simulink model "pvgrid"  (Simulink 7.8)
settings: Solver=ode23t  StartTime=0.0  StopTime=0.15  RelTol=1e-3
libraries: powerlib x15, powerlib_extras x5, simulink x1
settings Model: Creator=Administrator  LastModifiedBy=shinesong
settings OptimizationCC: InitFltsAndDblsToZero=on
settings DebuggingCC: FcnCallInpInsideContextMsg=Use local settings  StrictBusMsg=Warning

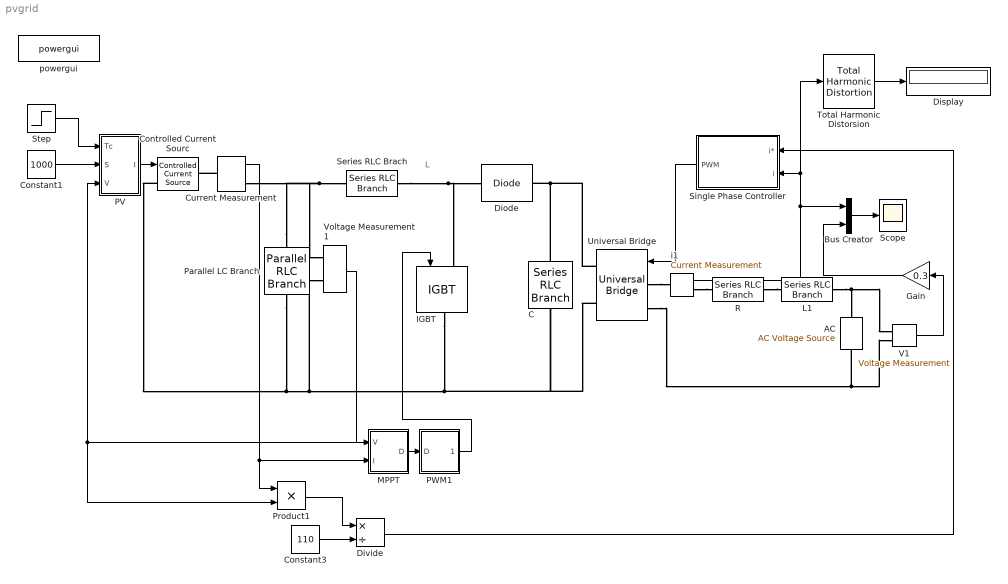
== system pvgrid ==
  note: L
  AC : powerlib/Electrical Sources/AC Voltage Source  Amplitude=155.5  Phase=0  Frequency=60  SampleTime=0  Measurements=None
  Bus Creator : BusCreator  Inputs=2
  C : powerlib/Elements/Series RLC Branch  LConnTagsString=__new0  RConnTagsString=__new0  BranchType=C  Resistance=1.0  Inductance=1.0  SetiL0=off  InitialCurrent=0  Capacitance=22e-6  Setx0=off  InitialVoltage=0  Measurements=None
  Constant1 : Constant  Value=1000
  Constant3 : Constant  Value=110
  Controlled Current Sourc : powerlib/Electrical Sources/Controlled Current Source  Initialize=on  Source_Type=DC  Amplitude=0  Phase=0  Frequency=0  Measurements=None
  Current Measurement : powerlib/Measurements/Current Measurement  PhasorSimulation=off  OutputType=Complex  PSBequivalent=0
  Diode : powerlib/Power Electronics/Diode  Ron=0.001  Lon=0  Vf=0.8  IC=0  UseSnubber=off  Rs=500  Cs=250e-9  Measurements=off
  Display : Display
  Divide : Product  Inputs=*/
  Gain : Gain  Gain=0.3
  IGBT : powerlib/Power Electronics/IGBT  Ron=0.001  Lon=0  Vf=1  Tf=1e-6  Tt=2e-6  IC=0  Rs=1e5  Cs=inf  Measurements=off
  L1 : powerlib/Elements/Series RLC Branch  LConnTagsString=__new0  RConnTagsString=__new0  BranchType=L  Resistance=1.0  Inductance=2e-2  SetiL0=off  InitialCurrent=0  Capacitance=1.0  Setx0=off  InitialVoltage=0  Measurements=None
  MPPT : Subsystem
  PV : Subsystem  mask{Im=13.88, Vm=281.6, Voc=353.6, Isc=14.88, Sref=1000, Tref=25, a=0.015, b=0.7, Rs=2}
      mask help: PV_modle
  PWM1 : Subsystem  mask{Ts=0.00001, Fs=5e4}
      mask prompts: Ts "Sample Time"; Fs "Frequency of Tri Wave"
  Parallel LC Branch : powerlib/Elements/Parallel RLC Branch  LConnTagsString=a  RConnTagsString=__new0  BranchType=C  Resistance=1.0  Inductance=1.0  SetiL0=off  InitialCurrent=0  Capacitance=110e-6  Setx0=off  InitialVoltage=0  Measurements=None
  Product1 : Product  RndMeth=Zero
  R : powerlib/Elements/Series RLC Branch  LConnTagsString=__new0  RConnTagsString=__new0  BranchType=R  Resistance=0.01  Inductance=10e-3  SetiL0=off  InitialCurrent=0  Capacitance=1.0  Setx0=off  InitialVoltage=0  Measurements=None
  Scope : Scope
      settings: YMin=2.5  YMax=35
  Series RLC Brach : powerlib/Elements/Series RLC Branch  LConnTagsString=__new0  RConnTagsString=__new0  BranchType=L  Resistance=1.0  Inductance=150e-6  SetiL0=off  InitialCurrent=0  Capacitance=1.0  Setx0=off  InitialVoltage=0  Measurements=None
  Single Phase Controller : Subsystem
  Step : Step  Time=0.1  Before=25  After=85  SampleTime=0
  Total Harmonic Distorsion : powerlib_extras/Measurements/Total Harmonic Distortion  f1=60
  Universal Bridge : powerlib/Power Electronics/Universal Bridge  Arms=2  SnubberResistance=1e5  SnubberCapacitance=inf  Device=MOSFET / Diodes  Ron=1e-3  Lon=0  ForwardVoltages="[  0  0  ]"  ForwardVoltage=0  GTOparameters=[ 10e-6 , 20e-6 ]  IGBTparameters=[ 1e-6 , 2e-6 ]  Measurements=None  Measurements_2=None  converterType=Rectifier
  V1 : powerlib/Measurements/Voltage Measurement  PhasorSimulation=off  OutputType=Complex  PSBequivalent=0
  Voltage Measurement1 : powerlib/Measurements/Voltage Measurement  PhasorSimulation=off  OutputType=Complex  PSBequivalent=0
  i1 : powerlib/Measurements/Current Measurement  PhasorSimulation=off  OutputType=Complex  PSBequivalent=0
  powergui : powerlib/powergui  SimulationMode=Discrete  SolverType=Tustin  SampleTime=5e-7  frequency=60  SPID=off  DisableSnubberDevices=off  DisableRonSwitches=off  DisableVfSwitches=off  SwTol=0  Interpol=off  DisplayEquations=off  FunctionMessages=off  frequencyindice=60  Pbase=100e6  ErrMax=1e-4  Iterations=50  UnitsV=kV  UnitsW=MW  echomessages=off  HookPort=off  EnableUseOfTLC=off  x0status=blocks  RestoreLinks=warning  ResistiveCurrentMeasurement=off  Frange=[0:2:500]  Ylog=off  Xlog=on  ShowGrid=off  save=off  variable=ZData  structure=ScopeData5  ZoomFFT=off  StartTime=0.0  cycles=1  DisplayStyle=1  fundamental=60  FreqAxis=off  MaxFrequency=1000  frequencyindicesteady=1  RmsSteady=1  display=off  Ts=0  methode=off
  wires:
  Single Phase Controller/1(PWM) -> Universal Bridge/1
  i1/1 -> Bus Creator/1, Single Phase Controller/2(i), Total Harmonic Distorsion/1
  Product1/1 -> Divide/1
  Voltage Measurement1/1 -> Product1/2, PV/3(V), MPPT/1(V)
  Constant3/1 -> Divide/2
  Divide/1 -> Single Phase Controller/1(i*)
  Bus Creator/1 -> Scope/1
  PV/1(I) -> Controlled Current Sourc/1
  Step/1 -> PV/1(Tc)
  MPPT/1(D) -> PWM1/1(D)
  Total Harmonic Distorsion/1 -> Display/1
  Current Measurement/1 -> Product1/1, MPPT/2(I)
  PWM1/1(pwm) -> IGBT/1
  Constant1/1 -> PV/2(S)
  V1/1 -> Gain/1
  Gain/1 -> Bus Creator/2
  connections:
  Universal Bridge/LConn1 -- i1/LConn1
  i1/RConn1 -- R/LConn1
  R/RConn1 -- L1/LConn1
  Universal Bridge/LConn2 -- AC/LConn1 -- V1/LConn2
  L1/RConn1 -- AC/RConn1 -- V1/LConn1
  Parallel LC Branch/LConn1 -- Current Measurement/RConn1 -- Voltage Measurement1/LConn1 -- Series RLC Brach/LConn1
  Series RLC Brach/RConn1 -- IGBT/LConn1 -- Diode/LConn1
  C/RConn1 -- IGBT/RConn1 -- Controlled Current Sourc/LConn1 -- Parallel LC Branch/RConn1 -- Voltage Measurement1/LConn2 -- Universal Bridge/RConn2
  C/LConn1 -- Diode/RConn1 -- Universal Bridge/RConn1
  Current Measurement/LConn1 -- Controlled Current Sourc/RConn1

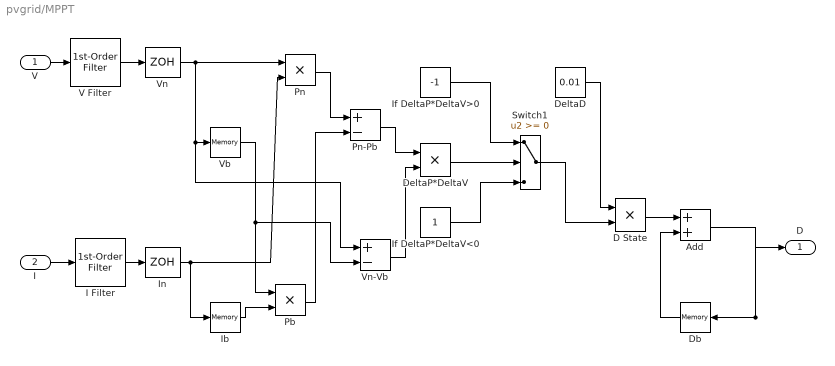
== system pvgrid/MPPT ==
  V : Inport
  I : Inport  Port=2
  Add : Sum
  D State : Product  RndMeth=Zero
  Db : Memory  InheritSampleTime=on  LinearizeAsDelay=on
  DeltaD : Constant  Value=0.01
  DeltaP*DeltaV : Product  RndMeth=Zero
  I Filter : powerlib_extras/Control  Blocks/1st-Order  Filter  FilterType=Lowpass  Tc=1e-3  Initialize=off  Vac_Init=[0.8 -25 60]  Vdc_Init=-0.4  PlotResponse=off  param1=[1 500 1]
  Ib : Memory  InheritSampleTime=on  LinearizeAsDelay=on
  If DeltaP*DeltaV<0 : Constant
  If DeltaP*DeltaV>0 : Constant  Value=-1
  In : ZeroOrderHold  SampleTime=1e-4
  Pb : Product  RndMeth=Zero
  Pn : Product  RndMeth=Zero
  Pn-Pb : Sum  Inputs=+-
  Switch1 : Switch
  V Filter : powerlib_extras/Control  Blocks/1st-Order  Filter  FilterType=Lowpass  Tc=1e-3  Initialize=off  Vac_Init=[0.8 -25 60]  Vdc_Init=-0.4  PlotResponse=off  param1=[1 500 1]
  Vb : Memory  InheritSampleTime=on  LinearizeAsDelay=on
  Vn : ZeroOrderHold  SampleTime=1e-4
  Vn-Vb : Sum  Inputs=+-
  D : Outport
  wires:
  V/1 -> V Filter/1
  I/1 -> I Filter/1
  V Filter/1 -> Vn/1
  I Filter/1 -> In/1
  In/1 -> Ib/1, Pn/2
  Vn/1 -> Pn/1, Vb/1, Vn-Vb/1
  Ib/1 -> Pb/2
  Vb/1 -> Pb/1, Vn-Vb/2
  Pn/1 -> Pn-Pb/1
  Pb/1 -> Pn-Pb/2
  D State/1 -> Add/1
  Add/1 -> Db/1, D/1
  Db/1 -> Add/2
  Pn-Pb/1 -> DeltaP*DeltaV/1
  Vn-Vb/1 -> DeltaP*DeltaV/2
  DeltaP*DeltaV/1 -> Switch1/2
  If DeltaP*DeltaV>0/1 -> Switch1/1
  If DeltaP*DeltaV<0/1 -> Switch1/3
  Switch1/1 -> D State/2
  DeltaD/1 -> D State/1

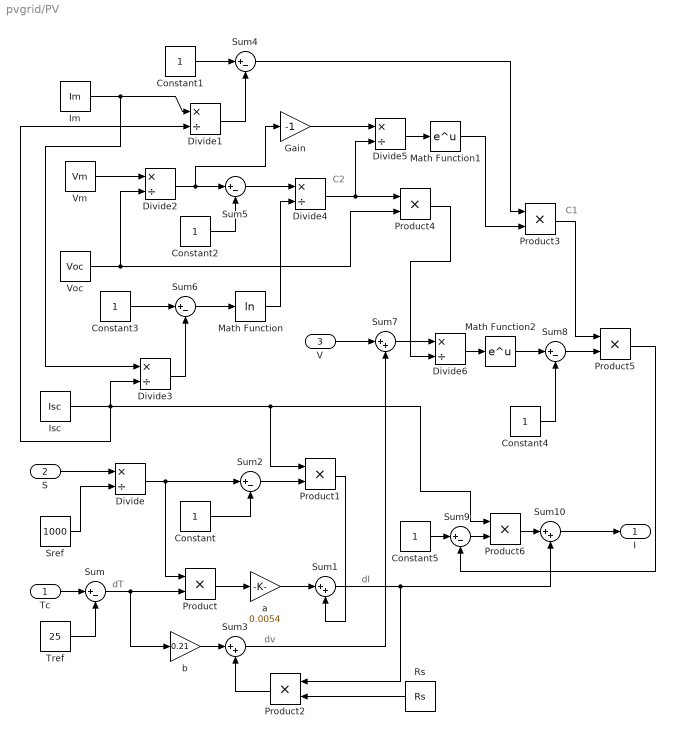
== system pvgrid/PV ==
  note: C2
  note: dI
  note: dv
  note: dT
  note: C1
  Tc : Inport
  S : Inport  Port=2
  V : Inport  Port=3
  Constant{,1..5} (6 alike) : Constant
  Divide{,1..6} (7 alike) : Product  Inputs=*/
  Gain : Gain  Gain=-1
  Im : Constant  Value=Im
  Isc : Constant  Value=Isc
  Math Function : Math  Operator=log  SaturateOnIntegerOverflow=on
  Math Function1 : Math  SaturateOnIntegerOverflow=on
  Math Function2 : Math  SaturateOnIntegerOverflow=on
  Product{,1..6} (7 alike) : Product  RndMeth=Zero
  Rs : Constant  Value=Rs
  Sref : Constant  Value=1000
  Sum{,2,4..6,8..9} (7 alike) : Sum  Inputs=|+-
  Sum{1,3,7,10} (4 alike) : Sum  Inputs=|++
  Tref : Constant  Value=25
  Vm : Constant  Value=Vm
  Voc : Constant  Value=Voc
  a : Gain  Gain=0.0054
  b : Gain  Gain=0.21
  I : Outport
  wires:
  Tc/1 -> Sum/1
  Tref/1 -> Sum/2
  Sum/1 -> Product/2, b/1
  S/1 -> Divide/1
  Sref/1 -> Divide/2
  Divide/1 -> Product/1, Sum2/1
  Product/1 -> a/1
  Constant/1 -> Sum2/2
  Sum2/1 -> Product1/2
  Product1/1 -> Sum1/2
  a/1 -> Sum1/1
  Sum1/1 -> Product2/1, Sum10/2
  b/1 -> Sum3/1
  Rs/1 -> Product2/2
  Product2/1 -> Sum3/2
  Sum3/1 -> Sum7/2
  Constant1/1 -> Sum4/1
  Im/1 -> Divide3/1, Divide1/1
  Divide1/1 -> Sum4/2
  Vm/1 -> Divide2/1
  Voc/1 -> Divide2/2, Product4/2
  Divide2/1 -> Sum5/1, Gain/1
  Constant2/1 -> Sum5/2
  Constant3/1 -> Sum6/1
  Divide3/1 -> Sum6/2
  Sum6/1 -> Math Function/1
  Sum5/1 -> Divide4/1
  Math Function/1 -> Divide4/2
  Divide4/1 -> Divide5/2, Product4/1
  Gain/1 -> Divide5/1
  Divide5/1 -> Math Function1/1
  Sum4/1 -> Product3/1
  Math Function1/1 -> Product3/2
  Product3/1 -> Product5/1
  Isc/1 -> Divide3/2, Product1/1, Divide1/2, Product6/1
  V/1 -> Sum7/1
  Sum7/1 -> Divide6/1
  Divide6/1 -> Math Function2/1
  Math Function2/1 -> Sum8/1
  Constant4/1 -> Sum8/2
  Sum8/1 -> Product5/2
  Constant5/1 -> Sum9/1
  Product5/1 -> Sum9/2
  Sum9/1 -> Product6/2
  Product6/1 -> Sum10/1
  Product4/1 -> Divide6/2
  Sum10/1 -> I/1

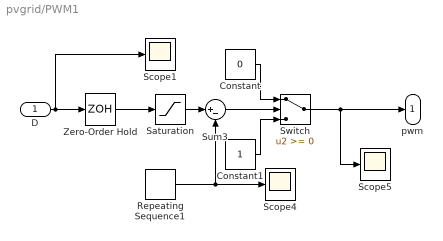
== system pvgrid/PWM1 ==
  D : Inport
  Constant : Constant  Value=0
  Constant1 : Constant
  Repeating Sequence1 : simulink/Sources/Repeating Sequence  rep_seq_t=[0 1/Fs/2 1/Fs]  rep_seq_y=[0 1 0]
  Saturation : Saturate  UpperLimit=0.6  LowerLimit=0.5
  Scope1 : Scope
      settings: YMin=0  YMax=3.25  SaveName=ScopeData7
  Scope4 : Scope
      settings: YMin=0.03825  YMax=0.0425  SaveName=ScopeData4
  Scope5 : Scope
      settings: YMin=0.95  YMax=1.05  SaveName=ScopeData5
  Sum3 : Sum  Inputs=|+-
  Switch : Switch
  Zero-Order Hold : ZeroOrderHold  SampleTime=Ts
  pwm : Outport
  wires:
  Saturation/1 -> Sum3/1
  Repeating Sequence1/1 -> Sum3/2, Scope4/1
  Sum3/1 -> Switch/2
  Constant1/1 -> Switch/3
  Constant/1 -> Switch/1
  Switch/1 -> Scope5/1, pwm/1
  D/1 -> Zero-Order Hold/1, Scope1/1
  Zero-Order Hold/1 -> Saturation/1

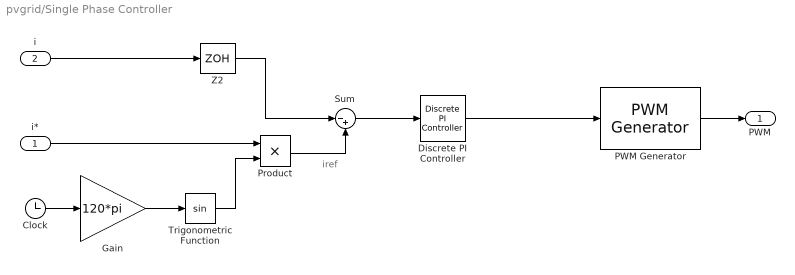
== system pvgrid/Single Phase Controller ==
  note: iref
  i* : Inport
  i : Inport  Port=2
  Clock : Clock
  Discrete PI Controller : powerlib_extras/Discrete  Control Blocks/Discrete PI Controller  Kp=6  Ki=256  Par_Limits=[1e6 -1e6]  Init=0  Ts=5e-7
  Gain : Gain  Gain=120*pi
  PWM Generator : powerlib_extras/Control  Blocks/PWM Generator  GeneratorMode="2-arm  bridge (4 pulses)"  Fc=5e3  Internal=off  mIndex=0.4  Freq=60  Phase=0
  Product : Product  RndMeth=Zero
  Sum : Sum  Inputs=|-+
  Trigonometric Function : Trigonometry
  Z2 : ZeroOrderHold  SampleTime=0.00001
  PWM : Outport
  wires:
  Gain/1 -> Trigonometric Function/1
  Trigonometric Function/1 -> Product/2
  Clock/1 -> Gain/1
  i*/1 -> Product/1
  i/1 -> Z2/1
  Z2/1 -> Sum/1
  Product/1 -> Sum/2
  Sum/1 -> Discrete PI Controller/1
  PWM Generator/1 -> PWM/1
  Discrete PI Controller/1 -> PWM Generator/1
